simulink model "Dynamic_articulation_FSF"  (R2018b)
settings: Solver=ode45  StartTime=0.0  StopTime=t_final  RelTol=1e-9
values from neighbouring files (symbols this model uses):
  A = [0 -1 0 0 0 0 0 0 ... (first row only)    [Dynamic_model_articulation.m]    (also in articulation1.m = E_matrix)
  a2 = input(12)    [Nonlinear_model.m]    (also in linear_model.m; linear_model_error.m; trailer_constants.m = 4.98)
  B1 = [0,B1(1),0,B1(2),0,B1(3),0,B1(4)]'    [articulation1.m]
  B2 = [0,B2(1),0,B2(2),0,B2(3),0,B2(4)]'    [articulation1.m]
  constants = [C1 C2 C3 m1 m2 I1 I2 a1 l1 h1 b1 a2 l2 Vx]    [Dynamic_model_articulation.m]
  h1 = input(10)    [Nonlinear_model.m]    (also in linear_model.m; linear_model_error.m; truck_constants.m = 1.1)
  K = place(A,B1,Poles)    [FullStateFeedback.m]    (also in articulation.m = [(C+C3),     (Cs1-C3*(h1+l2)+(m1+m2)*u^2),    (-C3*l2),    (; articulation1.m = [(C+C3),     (Cs1-C3*(h1+l2)+(m1+m2)*u^2),    (-C3*l2),    (; linear_model.m = -1/u*K*x_bar; linear_model_error.m = -1/u*K*x_bar)
  Vx = 20    [Dynamic_model_articulation.m]
settings Model: Creator=kevingasik  LastModifiedBy=kevingasik
settings SolverCC: ConsecutiveZCsStepRelTol=100*128*eps  MaxConsecutiveMinStep=10
settings DataIOCC: OutputOption=SpecifiedOutputTimes  OutputTimes=[0:0.04:t_final]

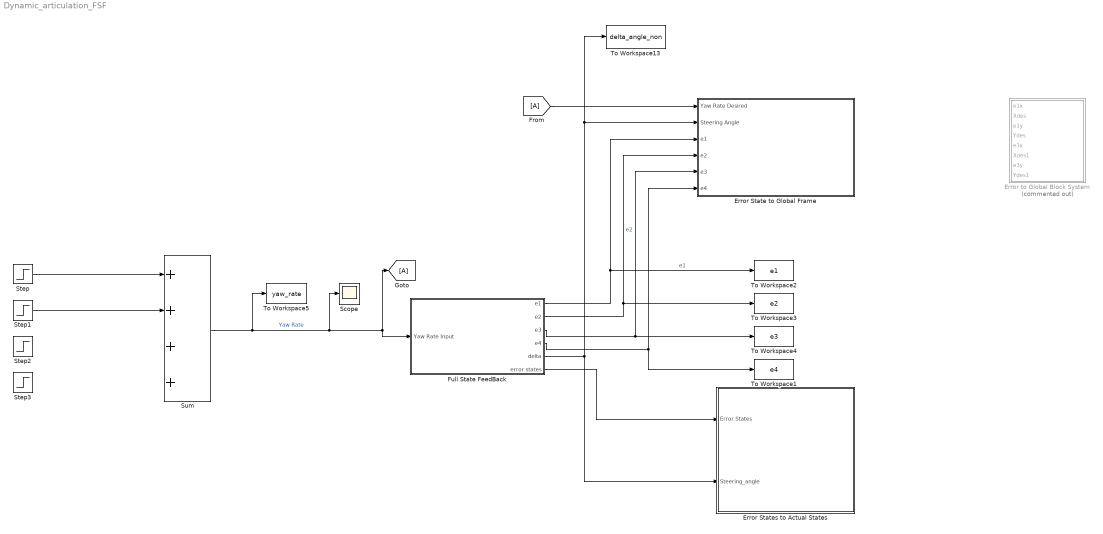
== system Dynamic_articulation_FSF ==
  Error State to Global Frame : Subsystem
  Error States to Actual States : Subsystem
  Error to Global Block System : Subsystem  Commented=on
  Full State FeedBack : Subsystem
  Scope : Scope
  Step : Step  Time=0  After=0  SampleTime=0
  Step1 : Step  Time=0  After=0.5/180*pi  SampleTime=0
  Step2 : Step  Time=200  After=-1/180*pi  SampleTime=0
  Step3 : Step  Time=110  After=0.5/180*pi  SampleTime=0
  Sum : Sum  Inputs=++++
  To Workspace1 : ToWorkspace  VariableName=e4  SampleTime=-1
      settings: Save2DSignal=2-D array (concatenate along first dimension)
  To Workspace13 : ToWorkspace  VariableName=delta_angle_non  SampleTime=-1
      settings: Save2DSignal=2-D array (concatenate along first dimension)
  To Workspace2 : ToWorkspace  VariableName=e1  SampleTime=-1
      settings: Save2DSignal=2-D array (concatenate along first dimension)
  To Workspace3 : ToWorkspace  VariableName=e2  SampleTime=-1
      settings: Save2DSignal=2-D array (concatenate along first dimension)
  To Workspace4 : ToWorkspace  VariableName=e3  SampleTime=-1
      settings: Save2DSignal=2-D array (concatenate along first dimension)
  To Workspace5 : ToWorkspace  VariableName=yaw_rate  SampleTime=-1
      settings: Save2DSignal=2-D array (concatenate along first dimension)
  wires:
  Sum/1 -> To Workspace5/1, [A], Full State FeedBack/1(Yaw Rate Input), Scope/1  "Yaw Rate"
  Full State FeedBack/2(e2) -> To Workspace3/1, Error State to Global Frame/4(e2)  "e2"
  Full State FeedBack/1(e1) -> Error State to Global Frame/3(e1), To Workspace2/1  "e1"
  Full State FeedBack/3(e3) -> Error State to Global Frame/5(e3), To Workspace4/1
  Full State FeedBack/4(e4) -> To Workspace1/1, Error State to Global Frame/6(e4)
  Full State FeedBack/5(delta) -> Error States to Actual States/2(Steering_angle), To Workspace13/1, Error State to Global Frame/2(Steering Angle)
  Step1/1 -> Sum/2
  Step/1 -> Sum/1
  [A] -> Error State to Global Frame/1(Yaw Rate Desired)
  Full State FeedBack/6(error states) -> Error States to Actual States/1(Error States)

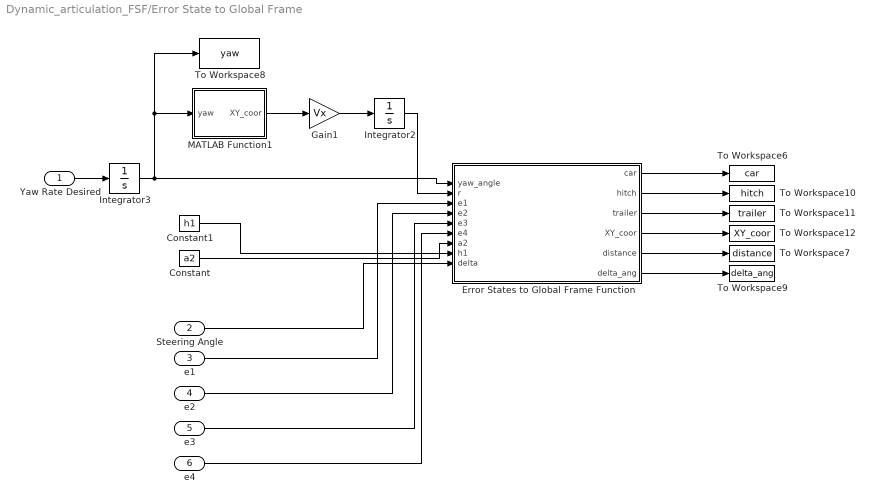
== system Dynamic_articulation_FSF/Error State to Global Frame ==
  Yaw Rate Desired : Inport
  Steering Angle : Inport  Port=2
  e1 : Inport  Port=3
  e2 : Inport  Port=4
  e3 : Inport  Port=5
  e4 : Inport  Port=6
  Constant : Constant  Value=a2
  Constant1 : Constant  Value=h1
  Error States to Global Frame Function : MATLAB Function  TreatAsAtomicUnit=on
  Gain1 : Gain  Gain=Vx
  Integrator2 : Integrator
  Integrator3 : Integrator
  MATLAB Function1 : MATLAB Function  TreatAsAtomicUnit=on
  To Workspace10 : ToWorkspace  VariableName=hitch  SampleTime=-1
      settings: Save2DSignal=2-D array (concatenate along first dimension)
  To Workspace11 : ToWorkspace  VariableName=trailer  SampleTime=-1
      settings: Save2DSignal=2-D array (concatenate along first dimension)
  To Workspace12 : ToWorkspace  VariableName=XY_coor  SampleTime=-1
      settings: Save2DSignal=2-D array (concatenate along first dimension)
  To Workspace6 : ToWorkspace  VariableName=car  SampleTime=-1
      settings: Save2DSignal=2-D array (concatenate along first dimension)
  To Workspace7 : ToWorkspace  VariableName=distance  SampleTime=-1
      settings: Save2DSignal=2-D array (concatenate along first dimension)
  To Workspace8 : ToWorkspace  VariableName=yaw  SampleTime=-1
      settings: Save2DSignal=2-D array (concatenate along first dimension)
  To Workspace9 : ToWorkspace  VariableName=delta_ang  SampleTime=-1
      settings: Save2DSignal=2-D array (concatenate along first dimension)
  wires:
  e4/1 -> Error States to Global Frame Function/6(e4)
  Error States to Global Frame Function/6(delta_ang) -> To Workspace9/1
  Yaw Rate Desired/1 -> Integrator3/1
  Error States to Global Frame Function/1(car) -> To Workspace6/1
  e2/1 -> Error States to Global Frame Function/4(e2)
  e1/1 -> Error States to Global Frame Function/3(e1)
  Gain1/1 -> Integrator2/1
  Error States to Global Frame Function/5(distance) -> To Workspace7/1
  Constant1/1 -> Error States to Global Frame Function/8(h1)
  e3/1 -> Error States to Global Frame Function/5(e3)
  MATLAB Function1/1(XY_coor) -> Gain1/1
  Error States to Global Frame Function/2(hitch) -> To Workspace10/1
  Integrator2/1 -> Error States to Global Frame Function/2(r)
  Steering Angle/1 -> Error States to Global Frame Function/9(delta)
  Constant/1 -> Error States to Global Frame Function/7(a2)
  Error States to Global Frame Function/4(XY_coor) -> To Workspace12/1
  Integrator3/1 -> MATLAB Function1/1(yaw), To Workspace8/1, Error States to Global Frame Function/1(yaw_angle)
  Error States to Global Frame Function/3(trailer) -> To Workspace11/1

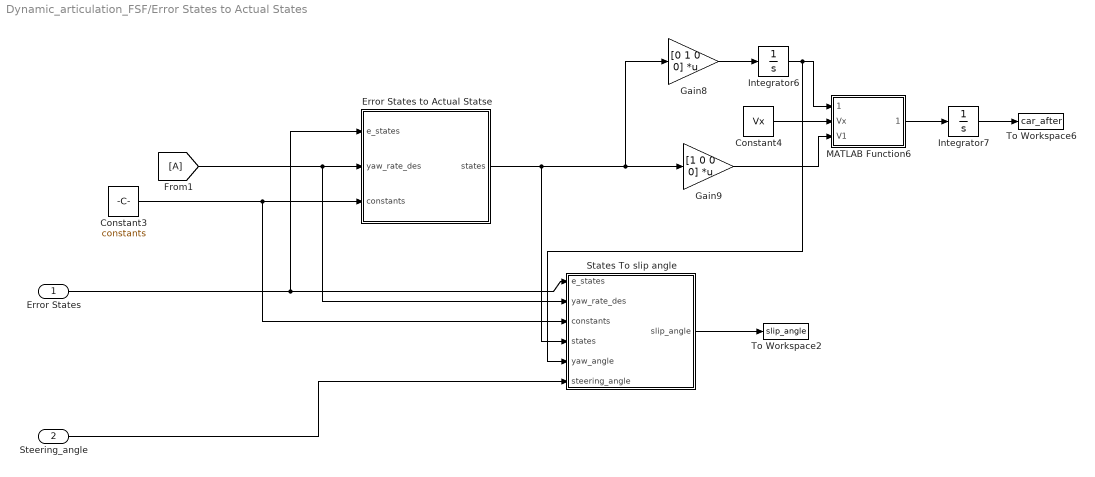
== system Dynamic_articulation_FSF/Error States to Actual States ==
  Error States : Inport
  Steering_angle : Inport  Port=2
  Constant3 : Constant  Value=constants
  Constant4 : Constant  Value=Vx
  Error States to Actual Statse : MATLAB Function  TreatAsAtomicUnit=on
  Gain8 : Gain  Gain=[0 1 0 0]  Multiplication=Matrix(K*u)
  Gain9 : Gain  Gain=[1 0 0 0]  Multiplication=Matrix(K*u)
  Integrator6 : Integrator
  Integrator7 : Integrator
  MATLAB Function6 : MATLAB Function  TreatAsAtomicUnit=on
  States To slip angle : MATLAB Function  TreatAsAtomicUnit=on
  To Workspace2 : ToWorkspace  VariableName=slip_angle  SampleTime=-1
      settings: Save2DSignal=2-D array (concatenate along first dimension)
  To Workspace6 : ToWorkspace  VariableName=car_after  SampleTime=-1
      settings: Save2DSignal=2-D array (concatenate along first dimension)
  wires:
  Constant3/1 -> States To slip angle/3(constants), Error States to Actual Statse/3(constants)
  Gain9/1 -> MATLAB Function6/3(V1)
  MATLAB Function6/1(XY_coor) -> Integrator7/1
  Error States/1 -> States To slip angle/1(e_states), Error States to Actual Statse/1(e_states)
  Constant4/1 -> MATLAB Function6/2(Vx)
  Error States to Actual Statse/1(states) -> States To slip angle/4(states), Gain9/1, Gain8/1
  Gain8/1 -> Integrator6/1
  Integrator7/1 -> To Workspace6/1
  [A] -> States To slip angle/2(yaw_rate_des), Error States to Actual Statse/2(yaw_rate_des)
  Steering_angle/1 -> States To slip angle/6(steering_angle)
  Integrator6/1 -> States To slip angle/5(yaw_angle), MATLAB Function6/1(yaw_angle)
  States To slip angle/1(slip_angle) -> To Workspace2/1

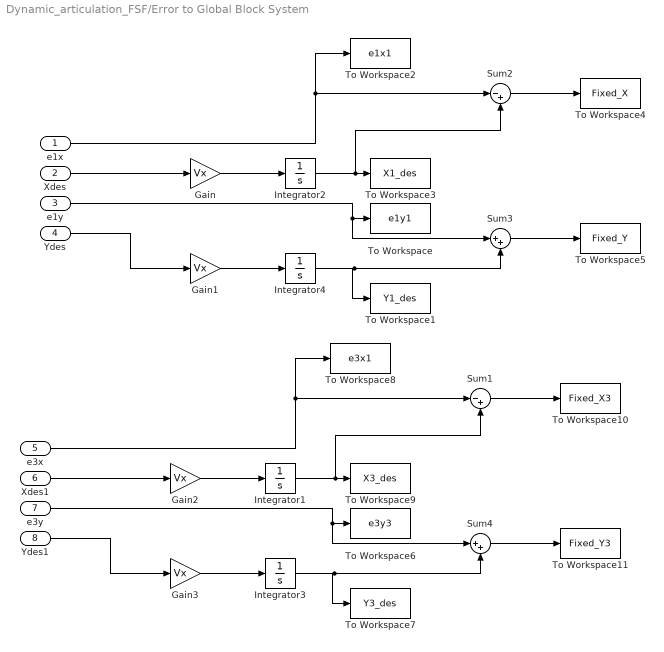
== system Dynamic_articulation_FSF/Error to Global Block System ==
  e1x : Inport
  Xdes : Inport  Port=2
  e1y : Inport  Port=3
  Ydes : Inport  Port=4
  e3x : Inport  Port=5
  Xdes1 : Inport  Port=6
  e3y : Inport  Port=7
  Ydes1 : Inport  Port=8
  Gain{,1..3} (4 alike) : Gain  Gain=Vx
  Integrator{1..4} (4 alike) : Integrator
  Sum1 : Sum  Inputs=|-+
  Sum2 : Sum  Inputs=|-+
  Sum3 : Sum  Inputs=|++
  Sum4 : Sum  Inputs=|++
  To Workspace : ToWorkspace  VariableName=e1y1  SampleTime=-1
      settings: Save2DSignal=2-D array (concatenate along first dimension)
  To Workspace1 : ToWorkspace  VariableName=Y1_des  SampleTime=-1
      settings: Save2DSignal=2-D array (concatenate along first dimension)
  To Workspace10 : ToWorkspace  VariableName=Fixed_X3  SampleTime=-1
      settings: Save2DSignal=2-D array (concatenate along first dimension)
  To Workspace11 : ToWorkspace  VariableName=Fixed_Y3  SampleTime=-1
      settings: Save2DSignal=2-D array (concatenate along first dimension)
  To Workspace2 : ToWorkspace  VariableName=e1x1  SampleTime=-1
      settings: Save2DSignal=2-D array (concatenate along first dimension)
  To Workspace3 : ToWorkspace  VariableName=X1_des  SampleTime=-1
      settings: Save2DSignal=2-D array (concatenate along first dimension)
  To Workspace4 : ToWorkspace  VariableName=Fixed_X  SampleTime=-1
      settings: Save2DSignal=2-D array (concatenate along first dimension)
  To Workspace5 : ToWorkspace  VariableName=Fixed_Y  SampleTime=-1
      settings: Save2DSignal=2-D array (concatenate along first dimension)
  To Workspace6 : ToWorkspace  VariableName=e3y3  SampleTime=-1
      settings: Save2DSignal=2-D array (concatenate along first dimension)
  To Workspace7 : ToWorkspace  VariableName=Y3_des  SampleTime=-1
      settings: Save2DSignal=2-D array (concatenate along first dimension)
  To Workspace8 : ToWorkspace  VariableName=e3x1  SampleTime=-1
      settings: Save2DSignal=2-D array (concatenate along first dimension)
  To Workspace9 : ToWorkspace  VariableName=X3_des  SampleTime=-1
      settings: Save2DSignal=2-D array (concatenate along first dimension)
  wires:
  Integrator4/1 -> To Workspace1/1, Sum3/2
  Xdes/1 -> Gain/1
  e1y/1 -> Sum3/1, To Workspace/1
  Gain1/1 -> Integrator4/1
  Sum3/1 -> To Workspace5/1
  Integrator2/1 -> Sum2/2, To Workspace3/1
  Gain/1 -> Integrator2/1
  e1x/1 -> To Workspace2/1, Sum2/1
  Sum2/1 -> To Workspace4/1
  Ydes/1 -> Gain1/1
  Sum1/1 -> To Workspace10/1
  Integrator1/1 -> Sum1/2, To Workspace9/1
  e3x/1 -> To Workspace8/1, Sum1/1
  Xdes1/1 -> Gain2/1
  e3y/1 -> Sum4/1, To Workspace6/1
  Gain3/1 -> Integrator3/1
  Sum4/1 -> To Workspace11/1
  Gain2/1 -> Integrator1/1
  Ydes1/1 -> Gain3/1
  Integrator3/1 -> To Workspace7/1, Sum4/2

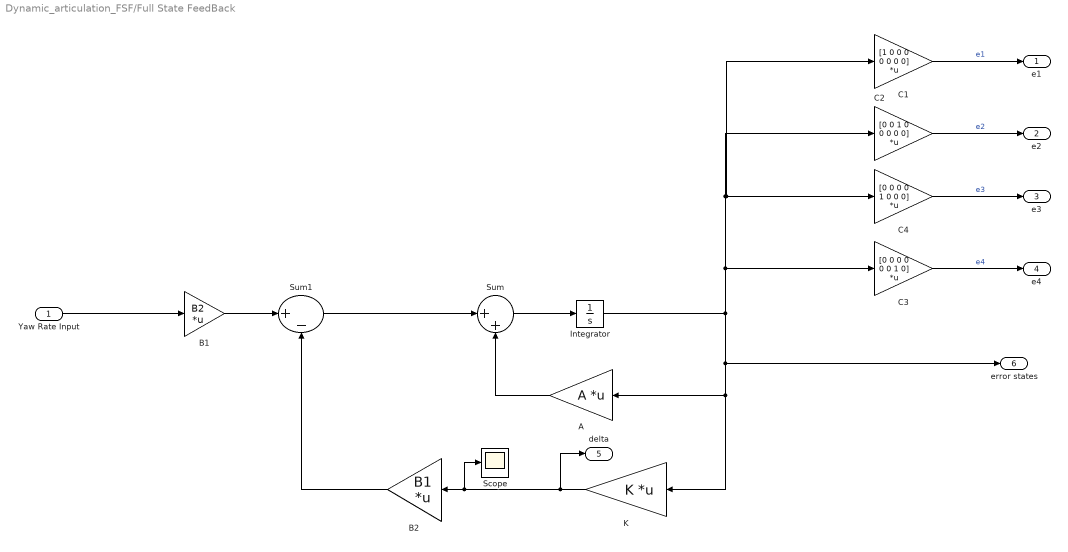
== system Dynamic_articulation_FSF/Full State FeedBack ==
  Yaw Rate Input : Inport
  A : Gain  Gain=A  Multiplication=Matrix(K*u)
  B1 : Gain  Gain=B2  Multiplication=Matrix(K*u)
  B2 : Gain  Gain=B1  Multiplication=Matrix(K*u)
  C1 : Gain  Gain=[1 0 0 0 0 0 0 0]  Multiplication=Matrix(K*u)
  C2 : Gain  Gain=[0 0 1 0 0 0 0 0]  Multiplication=Matrix(K*u)
  C3 : Gain  Gain=[0 0 0 0 0 0 1 0]  Multiplication=Matrix(K*u)
  C4 : Gain  Gain=[0 0 0 0 1 0 0 0]  Multiplication=Matrix(K*u)
  Integrator : Integrator  InitialCondition=0.0001
  K : Gain  Gain=K  Multiplication=Matrix(K*u)
  Scope : Scope
  Sum : Sum  Inputs=|++
  Sum1 : Sum  Inputs=|+-
  e1 : Outport
  e2 : Outport  Port=2
  e3 : Outport  Port=3
  e4 : Outport  Port=4
  delta : Outport  Port=5
  error states : Outport  Port=6
  wires:
  Sum/1 -> Integrator/1
  C2/1 -> e2/1  "e2"
  A/1 -> Sum/2
  C1/1 -> e1/1  "e1"
  C4/1 -> e3/1  "e3"
  C3/1 -> e4/1  "e4"
  K/1 -> Scope/1, B2/1, delta/1
  Integrator/1 -> error states/1, K/1, A/1, C2/1, C1/1, C4/1, C3/1
  Yaw Rate Input/1 -> B1/1
  B1/1 -> Sum1/1
  B2/1 -> Sum1/2
  Sum1/1 -> Sum/1

== matlab function Dynamic_articulation_FSF/Error State to Global Frame/Error States to Global Frame Function ==
  data: yaw_angle input; r input; e1 input; car output; hitch output; trailer output; XY_coor output; e2 input; e3 input; e4 input; a2 input; h1 input; distance output; delta input; delta_ang output
function [car,hitch,trailer,XY_coor,distance,delta_ang] = fcn(yaw_angle,r,e1,e2,e3, e4, a2,h1,delta)
XY_coor = [0 0];
trailer = [0 0];
hitch = [0 0];
car = [0 0];
angle = 0;


%%Transformation matrices from local to global coordinates
Q = [-sin(yaw_angle+e2),cos(yaw_angle+e2)];
R = [-cos(yaw_angle+e2),-sin(yaw_angle+e2)];
T = [-cos(yaw_angle+e4),-sin(yaw_angle+e4)];

%% desired trajectory
X_des = r(1,1);
Y_des = r(1,2);
%X_des2 = r(1,1) - (a2+h1)*cosd(yaw_angle+e2);
%Y_des2 = r(1,2) - (a2+h1)*sind(yaw_angle+e2);
XY_coor = [X_des,Y_des];

%outputting the correct output.
car_x = r(1,1)+ e1*Q(1,1);
car_y = r(1,2)+ e1*Q(1,2);
car = [car_x,car_y];

hitch_x = r(1,1) + e1*Q(1,1) + h1*R(1,1);
hitch_y = r(1,2) + e1*Q(1,2) + h1*R(1,2);
%hitch_a = X_des2 + e3*Q(1,1) - a2*T(1,1);
%hitch_b = Y_des2 + e3*Q(1,2) - a2*T(1,2);
hitch = [hitch_x,hitch_y];


trailer_x = r(1,1)+ (e1)*Q(1,1) + h1*R(1,1) + a2*T(1,1);
trailer_y = r(1,2)+ (e1)*Q(1,2) + h1*R(1,2) + a2*T(1,2);
%trailer_x = X_des2 + e3*Q(1,1);
%trailer_y = Y_des2 + e3*Q(1,2);

distance = sqrt((abs(hitch_x-trailer_x))^2 + abs(hitch_y-trailer_y)^2);
delta_ang = delta + e2 + yaw_angle; 
trailer = [trailer_x,trailer_y];

== matlab function Dynamic_articulation_FSF/Error State to Global Frame/MATLAB Function1 ==
  data: yaw input; XY_coor output
function XY_coor  = fcn(yaw)

XY_coor = [cos(yaw),sin(yaw)];

== matlab function Dynamic_articulation_FSF/Error States to Actual States/Error States to Actual Statse ==
  data: e_states input; yaw_rate_des input; constants input; states output
function states = fcn(e_states,yaw_rate_des,constants)

states = [0;0;0;0];

a2 = constants(12);
u =  constants(14);

e = [e_states(1) e_states(3) e_states(5) e_states(7)]';
ed = [e_states(2) e_states(4) e_states(6) e_states(8)]';


p1 = [1,        0,              0,      0;
      0,        1,              0,      0;
      1/a2,     0,           -1/a2,     0;  
      0,        0,              0,      0];
                
p2 = [0,        -u,      0,      0;
      0,         0,      0,      0;
      0,     -u/a2,      0,   u/a2;
      0,        -1,      0,      1]; %% phi = -e2 + e4
               
p3 = [0;1;0;0]; % \dot \psi desired 

%solves the 1st order states of the system, ydot, psidot, phidot and phi.
states = p1*ed + p2*e + p3*yaw_rate_des;

== matlab function Dynamic_articulation_FSF/Error States to Actual States/States To slip angle ==
  data: e_states input; yaw_rate_des input; constants input; slip_angle output; states input; yaw_angle input; steering_angle input
function slip_angle = fcn(e_states,yaw_rate_des,constants,states,yaw_angle,steering_angle)

slip_angle = 0;

a1 = constants(8);
a2 = constants(12);
u =  constants(14);

e = [e_states(1) e_states(3) e_states(5) e_states(7)]';
ed = [e_states(2) e_states(4) e_states(6) e_states(8)]';


slip_angle = steering_angle - states(2)*a1/u - yaw_angle;

== matlab function Dynamic_articulation_FSF/Error States to Actual States/MATLAB Function6 ==
  data: yaw_angle input; XY_coor output; Vx input; V1 input
function XY_coor  = fcn(yaw_angle,Vx,V1)

XY_coor = [(Vx*cos(yaw_angle) - V1*sin(yaw_angle)),(V1*cos(yaw_angle) + Vx*sin(yaw_angle))];
%xdot = XY_coor(1);
%ydot = XY_coor(2);

%xdot_p = xdot*cos(yaw_angle) - ydot*sin(yaw_angle); 
%ydot_p = xdot*sin(yaw_angle) + ydot*cos(yaw_angle);

%XY_coor = [xdot_p, ydot_p];
